simulink model "SimpleFeatureTriggerDetector"  (R2016b)
settings: Solver=FixedStepDiscrete  StartTime=0.0  StopTime=inf  FixedStep=sCoreParams.core.stepPeriod  RelTol=1e-3
undefined symbols (not defined in the file or in its folder): Low, sCoreParams, sCoreParams_decoders_txDetector_anyAll, sCoreParams_decoders_txDetector_detectChannelInds, sCoreParams_decoders_txDetector_nDetectionsRequested, sCoreParams_decoders_txDetector_ProbabilityOfStim, sCoreParams_decoders_txDetector_txRMS, sCoreParams_decoders_txDetector_txSign
libraries: dspswit3 x1
settings Model: DataTypeOverride=Double  MinMaxOverflowLogging=ForceOff  Creator=anish  LastModifiedBy=rzelmann
settings SolverCC: EnableConcurrentExecution=on
settings DataIOCC: SaveFormat=StructureWithTime  SignalLoggingSaveFormat=ModelDataLogs  SaveOutput=off  SignalLogging=off  DSMLogging=off  SaveTime=off
settings OptimizationCC: BlockReduction=off  ConditionallyExecuteInputs=off  DefaultParameterBehavior=Inlined  OptimizeBlockIOStorage=off  BufferReuse=off  GlobalBufferReuse=off  ExpressionFolding=off  LocalBlockOutputs=off  LifeSpan=inf
settings DebuggingCC: SignalRangeChecking=error  SaveWithParameterizedLinksMsg=none  MultiTaskDSMMsg=warning  MultiTaskCondExecSysMsg=none  AllowSymbolicDim=off  ModelReferenceSymbolNameMessage=none  StateNameClashWarn=warning  SFUnexpectedBacktrackingDiag=warning  SFNoUnconditionalDefaultTransitionDiag=warning  SFExecutionAtInitializationDiag=none
settings HardwareCC: ProdBitPerPointer=32  ProdBitPerSizeT=32  ProdBitPerPtrDiffT=32  ProdLargestAtomicFloat=None  ProdWordSize=32  ProdLongLongMode=on  ProdHWDeviceType=Generic->32-bit x86 compatible  TargetBitPerPointer=64  TargetLargestAtomicFloat=Float  TargetLongLongMode=on  TargetIntDivRoundTo=Zero  TargetEndianess=LittleEndian  TargetWordSize=64  TargetHWDeviceType=Intel->x86-64 (Windows64)
settings ModelReferenceCC: UpdateModelReferenceTargets=Force  ModelReferenceNumInstancesAllowed=Single  ModelReferencePassRootInputsByReference=off
settings RTWCC: SystemTargetFile=slrt.tlc  TemplateMakefile=slrt_default_tmf  Description=Simulink Real-Time  BuildConfiguration=Faster Runs  RTWCompilerOptimization=on
settings TargetCC: CodeReplacementLibrary=XPC_BLAS  ParMdlRefBuildCompliant=on  ConcurrentExecutionCompliant=on  GeneratePreprocessorConditionals=Use local settings  MatFileLogging=on  MATLABClassNameForMDSCustomization=xpcAperiodicCustomization
settings ConfigComp: CovMetricSettings=dw  CovHtmlReporting=on  CovSaveCumulativeToWorkspaceVar=on  CovSaveSingleToWorkspaceVar=on  CovExternalEMLEnable=off  CovSFcnEnable=off

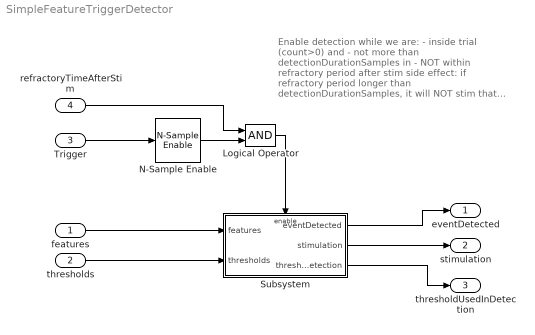
== system SimpleFeatureTriggerDetector ==
  note: Enable detection while we are:
      |  -  inside trial (count>0) and
      | - not more than detectionDurationSamples in
      | - NOT within refractory period after stim
      | side effect: if refractory period longer than detectionDurationSamples, it will NOT stim that next trial
  features : Inport  PortDimensions=[1 sCoreParams.decoders.txDetector.nFeatures]  SampleTime=sCoreParams.core.stepPeriod
  thresholds : Inport  Port=2  PortDimensions=[1 sCoreParams.decoders.txDetector.nFeatures]  SampleTime=sCoreParams.core.stepPeriod
  Trigger : Inport  Port=3  OutDataTypeStr=int32
  refractoryTimeAfterStim : Inport  Port=4  OutDataTypeStr=boolean  SampleTime=sCoreParams.core.stepPeriod
  Logical Operator : Logic  IconShape=distinctive  AllPortsSameDT=off  OutDataTypeStr=boolean
  N-Sample Enable : dspswit3/N-Sample Enable  N=sCoreParams.decoders.txDetector.detectionDurationSamples  ActiveLevel=Low (0)  reset=on  TriggerType=Non-zero sample  Ts=1  DataType=Logical
  Subsystem : Subsystem
  eventDetected : Outport  SampleTime=sCoreParams.core.stepPeriod
  stimulation : Outport  Port=2  SampleTime=sCoreParams.core.stepPeriod
  thresholdUsedInDetection : Outport  Port=3  SampleTime=sCoreParams.core.stepPeriod
  wires:
  features/1 -> Subsystem/1(features)
  thresholds/1 -> Subsystem/2(thresholds)
  Subsystem/1(eventDetected) -> eventDetected/1
  Subsystem/2(stimulation) -> stimulation/1
  Subsystem/3(thresholdUsedInDetection) -> thresholdUsedInDetection/1
  Trigger/1 -> N-Sample Enable/1
  Logical Operator/1 -> Subsystem/Enable
  refractoryTimeAfterStim/1 -> Logical Operator/1
  N-Sample Enable/1 -> Logical Operator/2

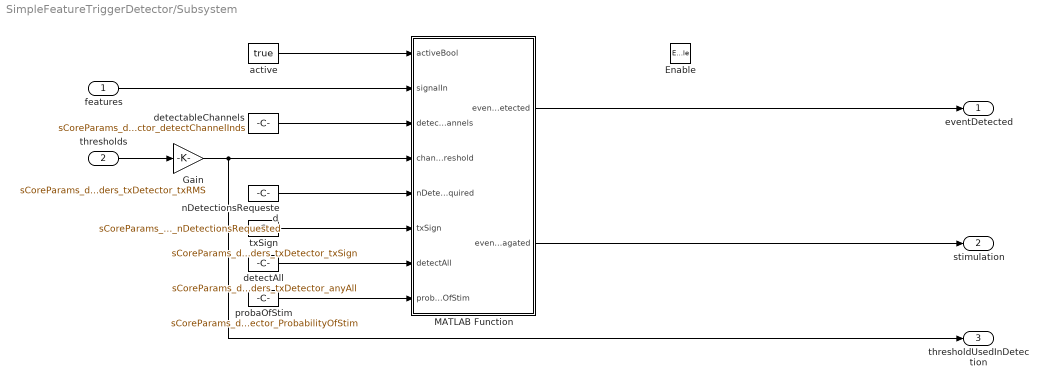
== system SimpleFeatureTriggerDetector/Subsystem ==
  features : Inport
  thresholds : Inport  Port=2
  Enable : EnablePort
  Gain : Gain  Gain=sCoreParams_decoders_txDetector_txRMS
  MATLAB Function : MATLAB Function  TreatAsAtomicUnit=on
  active : Constant  Value=true
  detectAll : Constant  Value=sCoreParams_decoders_txDetector_anyAll
  detectableChannels : Constant  Value=sCoreParams_decoders_txDetector_detectChannelInds
  nDetectionsRequested : Constant  Value=sCoreParams_decoders_txDetector_nDetectionsRequested
  probaOfStim : Constant  Value=sCoreParams_decoders_txDetector_ProbabilityOfStim
  txSign : Constant  Value=sCoreParams_decoders_txDetector_txSign
  eventDetected : Outport  OutputWhenDisabled=reset  InitialOutput=0
  stimulation : Outport  Port=2  InitialOutput=0
  thresholdUsedInDetection : Outport  Port=3
  wires:
  MATLAB Function/2(eventPropagated) -> stimulation/1
  Gain/1 -> thresholdUsedInDetection/1, MATLAB Function/4(channelThreshold)
  thresholds/1 -> Gain/1
  active/1 -> MATLAB Function/1(activeBool)
  nDetectionsRequested/1 -> MATLAB Function/5(nDetectionsRequired)
  MATLAB Function/1(eventDetected) -> eventDetected/1
  detectableChannels/1 -> MATLAB Function/3(detectableChannels)
  txSign/1 -> MATLAB Function/6(txSign)
  features/1 -> MATLAB Function/2(signalIn)
  detectAll/1 -> MATLAB Function/7(detectAll)
  probaOfStim/1 -> MATLAB Function/8(probabilityOfStim)

== matlab function SimpleFeatureTriggerDetector/Subsystem/MATLAB Function ==
  data: activeBool input; eventDetected output; signalIn input; detectableChannels input; channelThreshold input; nDetectionsRequired input; txSign input; eventPropagated output; detectAll input; probabilityOfStim input
function [eventDetected, eventPropagated] = TxThresholdCrossingDetector(activeBool, signalIn, detectableChannels, channelThreshold, nDetectionsRequired, txSign, detectAll, probabilityOfStim)
%#codegen

if (detectAll >= 1) % 1 means ALL - 0 means ANY
    [eventDetected, eventPropagated] = TxThresholdCrossingDetectorAll_EML(activeBool, signalIn, detectableChannels, channelThreshold, nDetectionsRequired, txSign, probabilityOfStim);
else % assumes ANY if detectAll is false
    [eventDetected, eventPropagated] = TxThresholdCrossingDetector_EML(activeBool, signalIn, detectableChannels, channelThreshold, nDetectionsRequired, txSign, probabilityOfStim);
end
